simulink model "Encoder"  (R2020b)
settings: Solver=VariableStepAuto  StartTime=0.0  StopTime=10.0  RelTol=1e-3
libraries: uavmavlinklib x1
settings Model: Creator=macra  LastModifiedBy=macra

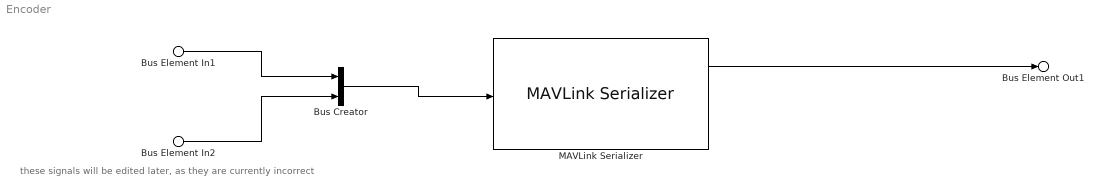
== system Encoder ==
  note: these signals will be edited later, as they are currently incorrect
  Bus Element In1 : Inport  PortName=Throttle Control
  Bus Element In2 : Inport  Port=2  PortName=Camera Control
  Bus Creator : BusCreator  Inputs=2
  MAVLink Serializer : uavmavlinklib/MAVLink Serializer  dialectSource=Select from standard MAVLink dialects  dialect=common.xml  dialectCustom=common.xml  version=2  messageType=HEARTBEAT
      settings: SourceProductBaseCode=UV
  Bus Element Out1 : Outport  PortName=Flight Command
  wires:
  Bus Element In1/1 -> Bus Creator/1
  Bus Element In2/1 -> Bus Creator/2
  Bus Creator/1 -> MAVLink Serializer/1
  MAVLink Serializer/1 -> Bus Element Out1/1
